simulink library "quat_norm"  (R2023b)
settings: Solver=VariableStepAuto  StartTime=0.0  StopTime=10.0  RelTol=1e-3
settings Model: Creator=robin  LastModifiedBy=robin

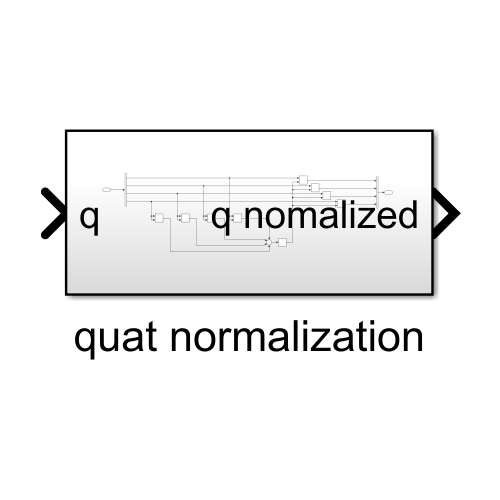
[thumbnail: Simulink's stored preview of the top-level diagram]
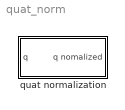
== system quat_norm ==
  quat normalization : Subsystem

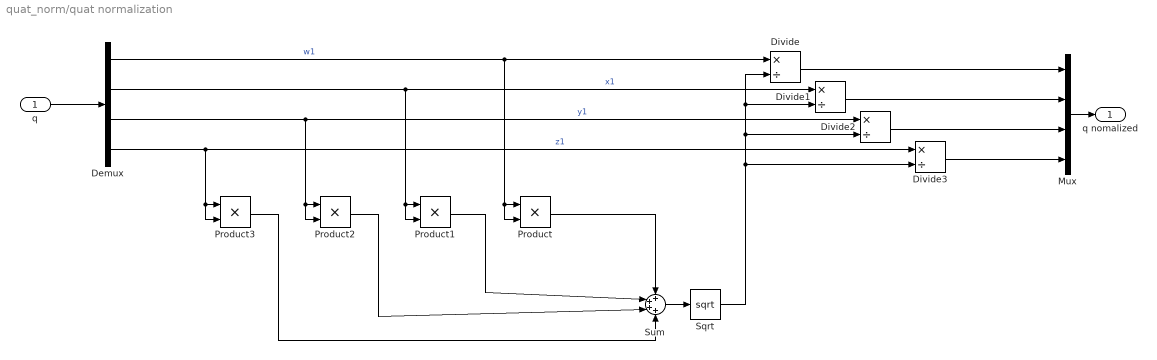
== system quat_norm/quat normalization ==
  q : Inport
  Demux : Demux
  Divide{,1..3} (4 alike) : Product  Inputs=*/
  Mux : Mux
  Product{,1..3} (4 alike) : Product
  Sqrt : Sqrt
  Sum : Sum  Inputs=++++
  q nomalized : Outport
  wires:
  Demux/1 -> Product/2, Product/1, Divide/1  "w1"
  Demux/2 -> Product1/2, Product1/1, Divide1/1  "x1"
  Demux/4 -> Product3/2, Product3/1, Divide3/1  "z1"
  Demux/3 -> Product2/2, Product2/1, Divide2/1  "y1"
  q/1 -> Demux/1
  Product/1 -> Sum/1
  Product1/1 -> Sum/2
  Product2/1 -> Sum/3
  Product3/1 -> Sum/4
  Sum/1 -> Sqrt/1
  Sqrt/1 -> Divide3/2, Divide2/2, Divide1/2, Divide/2
  Divide3/1 -> Mux/4
  Divide2/1 -> Mux/3
  Divide1/1 -> Mux/2
  Divide/1 -> Mux/1
  Mux/1 -> q nomalized/1
